simulink model "ex5_conv_interleaver"  (R2022a)
settings: Solver=FixedStepAuto  StartTime=0  StopTime=2  RelTol=1e-3
model workspace (MAT data in the model file):
  ITV_I = 12
  ITV_M = 17
  M = 4
  RS_k = 188
  RS_m = 8
  RS_n = 204
  RS_prim_poly = 'X^8+X^4+X^3+X^2+1'
  Rb = 1000
  SCR_init = [1 0 0 1 0 1 0 1 0 0 0 0 0 0 0]
  SCR_poly = '1+z^-14+z^-15'
  beta = 0.3
  osf = 16
  span = 12
libraries: commcnvintrlv2 x2, commsink2 x1, commrandsrc3 x1
settings Model: Creator=root  LastModifiedBy=Filippo
settings SolverCC: AlgebraicLoopSolver=TrustRegion
settings DataIOCC: ReturnWorkspaceOutputs=off
settings DebuggingCC: UnconnectedInputMsg=warning  UnconnectedOutputMsg=warning  UnconnectedLineMsg=warning  SFMachineParentedDataDiag=warning  ArithmeticOperatorsInVariantConditions=warning
settings SFSimCC: SimUseLocalCustomCode=off  CustomCodeUndefinedFunction=UseInterfaceOnly
settings RTWCC: RTWUseLocalCustomCode=off
settings CodeAppCC: StateflowObjectComments=on

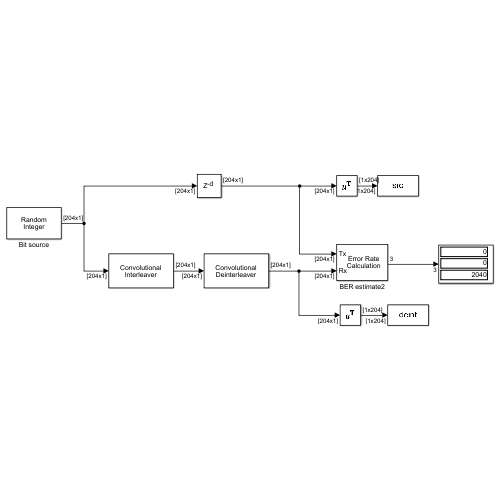
[thumbnail: Simulink's stored preview of the top-level diagram]
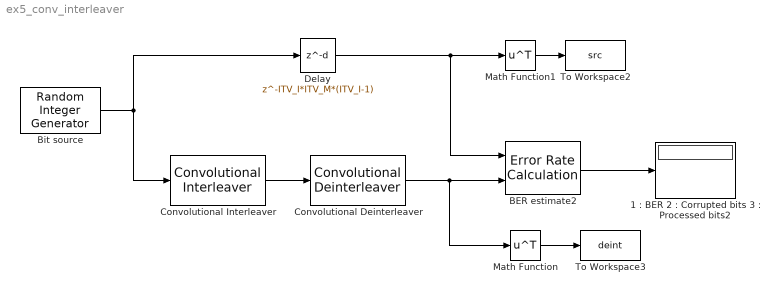
== system ex5_conv_interleaver ==
  "1 : BER 2 : Corrupted bits 3 : Processed bits2" : Display
  BER estimate2 : commsink2/Error Rate Calculation  N=0  st_delay=0  cp_mode=Entire frame  subframe=[]  PMode=Port  WsName=ErrorVec  RsMode2=off  stop=off  numErr=100  maxBits=1e6
  Bit source : commrandsrc3/Random Integer Generator  SetSize=2  SeedSource=Auto  Seed=1922  SampleTime=1/Rb  SamplesPerFrame=ITV_I*ITV_M  OutputDataType=uint8  SimulateUsing=Code generation
  Convolutional Deinterleaver : commcnvintrlv2/Convolutional Deinterleaver  N=ITV_I  B=ITV_M  ic=0
      settings: SourceProductBaseCode=CM
  Convolutional Interleaver : commcnvintrlv2/Convolutional Interleaver  N=ITV_I  B=ITV_M  ic=0
      settings: SourceProductBaseCode=CM
  Delay : Delay  DelayLength=ITV_I*ITV_M*(ITV_I-1)  InitialCondition=0  InputProcessing=Columns as channels (frame based)
  Math Function : Math  Operator=transpose
  Math Function1 : Math  Operator=transpose
  To Workspace2 : ToWorkspace  VariableName=src  SaveFormat=Timeseries  SampleTime=-1
  To Workspace3 : ToWorkspace  VariableName=deint  SaveFormat=Timeseries  SampleTime=-1
  wires:
  Convolutional Interleaver/1 -> Convolutional Deinterleaver/1
  BER estimate2/1 -> "1 : BER 2 : Corrupted bits 3 : Processed bits2"/1
  Convolutional Deinterleaver/1 -> Math Function/1, BER estimate2/2
  Delay/1 -> BER estimate2/1, Math Function1/1
  Math Function/1 -> To Workspace3/1
  Math Function1/1 -> To Workspace2/1
  Bit source/1 -> Delay/1, Convolutional Interleaver/1
